simulink model "ece456hw73"  (R2017b)
settings: Solver=VariableStepAuto  StartTime=0.0  StopTime=10.0  RelTol=1e-3
values from neighbouring files (symbols this model uses):
  tau = 35.35    [ece456hw6.m]    (also in ece456hw7.m = 1; ece456hw8.m = 1)
settings Model: Creator=b  LastModifiedBy=b

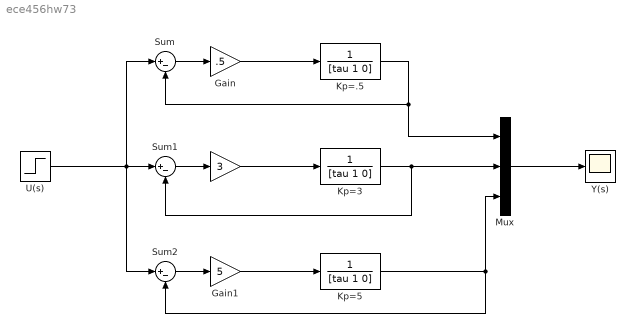
== system ece456hw73 ==
  " " : Gain  Gain=3
  Gain : Gain  Gain=.5
  Gain1 : Gain  Gain=5
  Kp=.5 : TransferFcn  Denominator=[tau 1 0]
  Kp=3 : TransferFcn  Denominator=[tau 1 0]
  Kp=5 : TransferFcn  Denominator=[tau 1 0]
  Mux : Mux  Inputs=3
  Sum : Sum  Inputs=|+-
  Sum1 : Sum  Inputs=|+-
  Sum2 : Sum  Inputs=|+-
  U(s) : Step  SampleTime=0
  Y(s) : Scope
  wires:
  U(s)/1 -> Sum2/1, Sum1/1, Sum/1
  Gain1/1 -> Kp=5/1
  Gain/1 -> Kp=.5/1
  Kp=.5/1 -> Sum/2, Mux/1
  Kp=5/1 -> Sum2/2, Mux/3
  " "/1 -> Kp=3/1
  Kp=3/1 -> Sum1/2, Mux/2
  Sum/1 -> Gain/1
  Sum1/1 -> " "/1
  Sum2/1 -> Gain1/1
  Mux/1 -> Y(s)/1
